simulink model "MySusp_DamperSystem_RTW"  (R2022a)
settings: Solver=ode1  StartTime=0.0  StopTime=inf  FixedStep=0.001  RelTol=1e-3
PreLoadFcn:
  | vehicle = 'Car'; if ~length(which('cmself')), cmenv; end
  | MySusp_DamperSystem_RTW_bus
  | MySusp_DamperSystem_RTW_params
InitFcn:
  | vehicle = 'Car'; if ~length(which('cmself')), cmenv; end
  | MySusp_DamperSystem_RTW_bus
undefined symbols (not defined in the file or in its folder): Damping_Pull_FL, Damping_Pull_FR, Damping_Pull_RL, Damping_Pull_RR, Damping_Push_FL, Damping_Push_FR, Damping_Push_RL, Damping_Push_RR
Description:
  | CarMaker Plug-in Model Target
settings Model: ModifiedByFormat=IPG  Creator=IPG  LastModifiedBy=IPG
settings SolverCC: AlgebraicLoopSolver=TrustRegion
settings DebuggingCC: UnconnectedInputMsg=warning  UnconnectedOutputMsg=warning  UnconnectedLineMsg=warning
settings RTWCC: Description=CarMaker Plug-in Model Target  SystemTargetFile=CarMaker.tlc  TemplateMakefile=CarMaker_unix-win64.tmf  DLArmComputeVersion=19.05
settings CodeAppCC: MaxIdLength=127
settings STFCustomTargetCC: TargetLangStandard=C99 (ISO)  CombineOutputUpdateFcns=on  MatFileLogging=on  CodeInterfacePackaging=Reusable function  GRTInterface=off  GenerateAllocFcn=on  SystemTargetFile=CarMaker.tlc
settings GRTTargetCC: ParMdlRefBuildCompliant=off  CompOptLevelCompliant=off  ConcurrentExecutionCompliant=off  CodeInterfacePackaging=Reusable function  CPPClassGenCompliant=off  GenerateAllocFcn=on  UseToolchainInfoCompliant=off

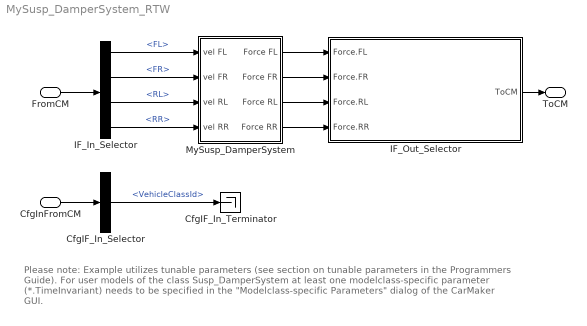
== system MySusp_DamperSystem_RTW ==
  note: Please note: Example utilizes tunable parameters (see section on tunable parameters in the Programmers Guide).
      |
      | For user models of the class Susp_DamperSystem at least one modelclass-specific parameter (*.TimeInvariant) needs to be
      | specified in the "Modelclass-specific Parameters" dialog of the CarMaker GUI.
  FromCM : Inport  OutDataTypeStr=Bus: cmSusp_DamperSystemIn
  CfgInFromCM : Inport  Port=2  OutDataTypeStr=Bus: cmSusp_DamperSystemCfgIn
  CfgIF_In_Selector : BusSelector  OutputSignals=VehicleClassId
  CfgIF_In_Terminator : Terminator
  IF_In_Selector : BusSelector  OutputSignals=vel.FL,vel.FR,vel.RL,vel.RR
  IF_Out_Selector : Subsystem  mask(Signal Selection){}
      mask help: Signal Selection Block
      settings: OpenFcn=cmSignalSelect('SignalSelection_CB',gcb)
  MySusp_DamperSystem : Subsystem
  ToCM : Outport  OutDataTypeStr=Bus: cmSusp_DamperSystemOut
  wires:
  FromCM/1 -> IF_In_Selector/1
  IF_Out_Selector/1(ToCM) -> ToCM/1
  CfgInFromCM/1 -> CfgIF_In_Selector/1
  CfgIF_In_Selector/1 -> CfgIF_In_Terminator/1  "<VehicleClassId>"
  MySusp_DamperSystem/1(Force FL) -> IF_Out_Selector/1(Force.FL)
  MySusp_DamperSystem/2(Force FR) -> IF_Out_Selector/2(Force.FR)
  MySusp_DamperSystem/3(Force RL) -> IF_Out_Selector/3(Force.RL)
  MySusp_DamperSystem/4(Force RR) -> IF_Out_Selector/4(Force.RR)
  IF_In_Selector/1 -> MySusp_DamperSystem/1(vel FL)  "<FL>"
  IF_In_Selector/2 -> MySusp_DamperSystem/2(vel FR)  "<FR>"
  IF_In_Selector/3 -> MySusp_DamperSystem/3(vel RL)  "<RL>"
  IF_In_Selector/4 -> MySusp_DamperSystem/4(vel RR)  "<RR>"

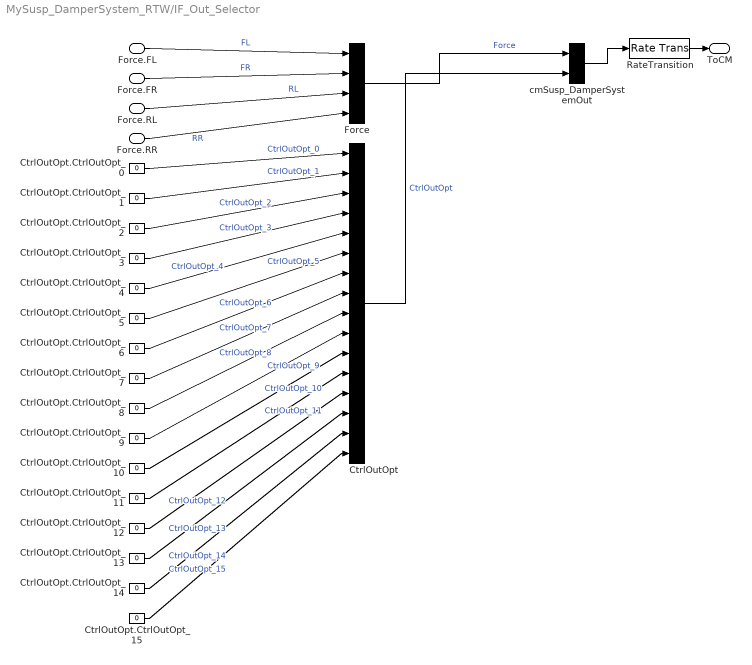
== system MySusp_DamperSystem_RTW/IF_Out_Selector ==
  Force.FL : Inport
  Force.FR : Inport  Port=2
  Force.RL : Inport  Port=3
  Force.RR : Inport  Port=4
  CtrlOutOpt : BusCreator  Inputs=16
  CtrlOutOpt.CtrlOutOpt_{0..15} (16 alike) : Constant  Value=0
  Force : BusCreator  Inputs=4
  RateTransition : RateTransition  OutPortSampleTime=str2num(get_param(bdroot,'FixedStep'))
  cmSusp_DamperSystemOut : BusCreator  Inputs=2
  ToCM : Outport
  wires:
  RateTransition/1 -> ToCM/1
  cmSusp_DamperSystemOut/1 -> RateTransition/1
  Force/1 -> cmSusp_DamperSystemOut/1  "Force"
  CtrlOutOpt/1 -> cmSusp_DamperSystemOut/2  "CtrlOutOpt"
  CtrlOutOpt.CtrlOutOpt_0/1 -> CtrlOutOpt/1  "CtrlOutOpt_0"
  CtrlOutOpt.CtrlOutOpt_1/1 -> CtrlOutOpt/2  "CtrlOutOpt_1"
  CtrlOutOpt.CtrlOutOpt_2/1 -> CtrlOutOpt/3  "CtrlOutOpt_2"
  CtrlOutOpt.CtrlOutOpt_3/1 -> CtrlOutOpt/4  "CtrlOutOpt_3"
  CtrlOutOpt.CtrlOutOpt_4/1 -> CtrlOutOpt/5  "CtrlOutOpt_4"
  CtrlOutOpt.CtrlOutOpt_5/1 -> CtrlOutOpt/6  "CtrlOutOpt_5"
  CtrlOutOpt.CtrlOutOpt_6/1 -> CtrlOutOpt/7  "CtrlOutOpt_6"
  CtrlOutOpt.CtrlOutOpt_7/1 -> CtrlOutOpt/8  "CtrlOutOpt_7"
  CtrlOutOpt.CtrlOutOpt_8/1 -> CtrlOutOpt/9  "CtrlOutOpt_8"
  CtrlOutOpt.CtrlOutOpt_9/1 -> CtrlOutOpt/10  "CtrlOutOpt_9"
  CtrlOutOpt.CtrlOutOpt_10/1 -> CtrlOutOpt/11  "CtrlOutOpt_10"
  CtrlOutOpt.CtrlOutOpt_11/1 -> CtrlOutOpt/12  "CtrlOutOpt_11"
  CtrlOutOpt.CtrlOutOpt_12/1 -> CtrlOutOpt/13  "CtrlOutOpt_12"
  CtrlOutOpt.CtrlOutOpt_13/1 -> CtrlOutOpt/14  "CtrlOutOpt_13"
  CtrlOutOpt.CtrlOutOpt_14/1 -> CtrlOutOpt/15  "CtrlOutOpt_14"
  CtrlOutOpt.CtrlOutOpt_15/1 -> CtrlOutOpt/16  "CtrlOutOpt_15"
  Force.FL/1 -> Force/1  "FL"
  Force.FR/1 -> Force/2  "FR"
  Force.RL/1 -> Force/3  "RL"
  Force.RR/1 -> Force/4  "RR"

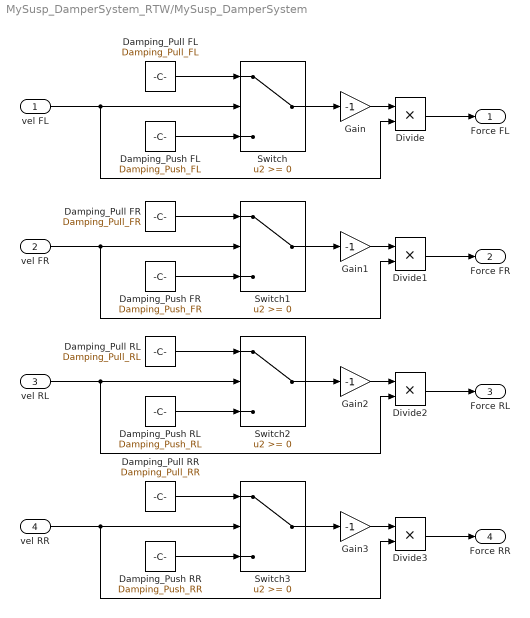
== system MySusp_DamperSystem_RTW/MySusp_DamperSystem ==
  vel FL : Inport
  vel FR : Inport  Port=2
  vel RL : Inport  Port=3
  vel RR : Inport  Port=4
  Damping_Pull FL : Constant  Value=Damping_Pull_FL
  Damping_Pull FR : Constant  Value=Damping_Pull_FR
  Damping_Pull RL : Constant  Value=Damping_Pull_RL
  Damping_Pull RR : Constant  Value=Damping_Pull_RR
  Damping_Push FL : Constant  Value=Damping_Push_FL
  Damping_Push FR : Constant  Value=Damping_Push_FR
  Damping_Push RL : Constant  Value=Damping_Push_RL
  Damping_Push RR : Constant  Value=Damping_Push_RR
  Divide{,1..3} (4 alike) : Product  Inputs=**
  Gain{,1..3} (4 alike) : Gain  Gain=-1
  Switch{,1..3} (4 alike) : Switch  SaturateOnIntegerOverflow=off  InputSameDT=off
  Force FL : Outport  VectorParamsAs1DForOutWhenUnconnected=off
  Force FR : Outport  Port=2  VectorParamsAs1DForOutWhenUnconnected=off
  Force RL : Outport  Port=3  VectorParamsAs1DForOutWhenUnconnected=off
  Force RR : Outport  Port=4  VectorParamsAs1DForOutWhenUnconnected=off
  wires:
  vel FL/1 -> Divide/2, Switch/2
  Switch/1 -> Gain/1
  Damping_Pull FL/1 -> Switch/1
  Damping_Push FL/1 -> Switch/3
  Gain/1 -> Divide/1
  Divide/1 -> Force FL/1
  Gain1/1 -> Divide1/1
  vel FR/1 -> Divide1/2, Switch1/2
  Switch1/1 -> Gain1/1
  Divide1/1 -> Force FR/1
  Damping_Pull FR/1 -> Switch1/1
  Damping_Push FR/1 -> Switch1/3
  Damping_Push RL/1 -> Switch2/3
  vel RL/1 -> Divide2/2, Switch2/2
  Damping_Pull RL/1 -> Switch2/1
  Switch2/1 -> Gain2/1
  Divide2/1 -> Force RL/1
  Gain2/1 -> Divide2/1
  Damping_Push RR/1 -> Switch3/3
  vel RR/1 -> Divide3/2, Switch3/2
  Damping_Pull RR/1 -> Switch3/1
  Switch3/1 -> Gain3/1
  Divide3/1 -> Force RR/1
  Gain3/1 -> Divide3/1
